simulink model "AntiBrake_model"  (R2019b)
settings: Solver=VariableStepAuto  StartTime=0.0  StopTime=20  MaxStep=0.001  RelTol=1e-3
InitFcn:
  | Cyclist_weight=85;
  | Vehicle_mass = 0.25; %Tire weight= 250g
  | gr = 9.81;
  | Wheel_Inertia = 0.0064;
  | Wheel_Radius = 0.3;
  | V=6.95; % in m/s
  | Effective_Radius_of_Disc = 0.16;
  | Coefficient_of_Brake_friction = 0.9;
  | pb=200;
  | Number_of_brake_pad = 1;
  | TB =0.01;
  | Abs=1;
libraries: simulink x1
settings Model: Creator=Avmash  LastModifiedBy=Avmash

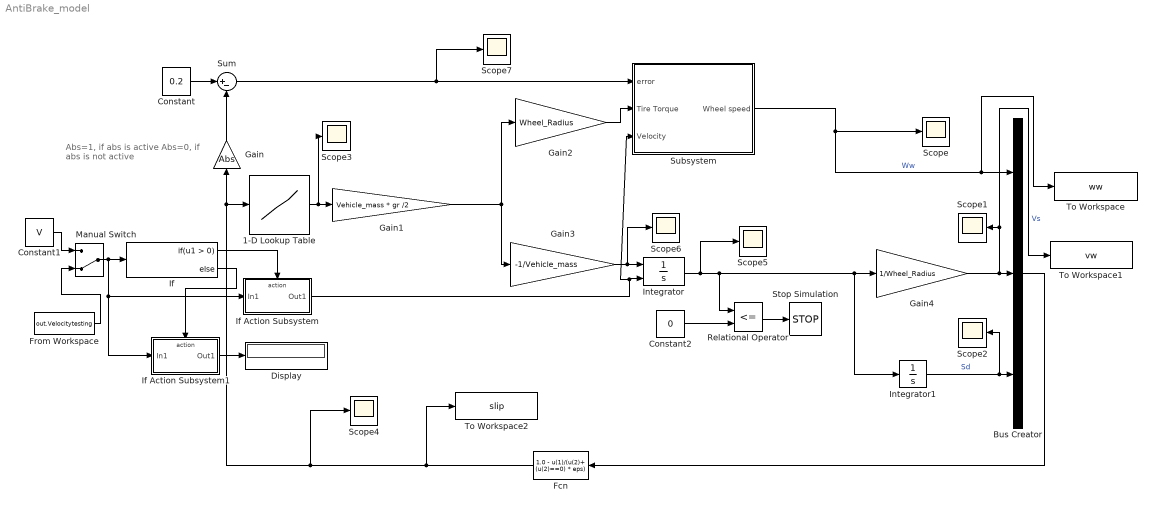
== system AntiBrake_model ==
  note: Abs=1, if abs is active
      | Abs=0, if abs is not active
  1-D Lookup Table : Lookup_n-D  NumberOfTableDimensions=1  BreakpointsForDimension1="[0\t0.0500000000000000\t0.100000000000000\t0.150000000000000\t0.200000000000000\t0.250000000000000\t0.300000000000000\t0.350000000000000\t0.400000000000000\t0.450000000000000\t0.500000000000000\t0.550000000000000\t0.600000000000000\t0.650000000000000\t0.700000000000000\t0.750000000000000\t0.800000000000000\t0.850000000000000\t0.900000000000000\t0.950000000000000\t1]"  Table="[0\t0.400000000000000\t0.800000000000000\t0.970000000000000\t1\t0.980000000000000\t0.960000000000000\t0.940000000000000\t0.920000000000000\t0.900000000000000\t0.880000000000000\t0.855000000000000\t0.830000000000000\t0.810000000000000\t0.790000000000000\t0.770000000000000\t0.750000000000000\t0.730000000000000\t0.720000000000000\t0.710000000000000\t0.700000000000000]"  InternalRulePriority=Speed  RndMeth=Simplest  InputSameDT=on
  Bus Creator : BusCreator  Inputs=3
  Constant : Constant  Value=0.2
  Constant1 : Constant  Value=V
  Constant2 : Constant  Value=0
  Display : Display
  Fcn : Fcn  Expr=1.0 - u(1)/(u(2)+ (u(2)==0) * eps)
  From Workspace : FromWorkspace  VariableName=out.Velocitytesting  SampleTime=0
  Gain : Gain  Gain=Abs
  Gain1 : Gain  Gain=Vehicle_mass * gr /2
  Gain2 : Gain  Gain=Wheel_Radius
  Gain3 : Gain  Gain=-1/Vehicle_mass
  Gain4 : Gain  Gain=1/Wheel_Radius
  If : If
  If Action Subsystem : Subsystem  TreatAsAtomicUnit=on
  If Action Subsystem1 : Subsystem  TreatAsAtomicUnit=on
  Integrator : Integrator  InitialConditionSource=external  InitialCondition=V  LimitOutput=on  UpperSaturationLimit=1000  LowerSaturationLimit=0
  Integrator1 : Integrator
  Manual Switch : ManualSwitch  CurrentSetting=0
  Relational Operator : RelationalOperator  Operator=<=  OutDataTypeStr=boolean  RndMeth=Simplest
  Scope{,1..7} (8 alike) : Scope
  Stop Simulation : Stop
  Subsystem : Subsystem
  Sum : Sum  Inputs=|+-
  To Workspace : ToWorkspace  VariableName=ww  SaveFormat=Timeseries  SampleTime=-1
  To Workspace1 : ToWorkspace  VariableName=vw  SaveFormat=Timeseries  SampleTime=-1
  To Workspace2 : ToWorkspace  VariableName=slip  SaveFormat=Timeseries  SampleTime=-1
  wires:
  1-D Lookup Table/1 -> Scope3/1, Gain1/1
  Constant/1 -> Sum/1
  Sum/1 -> Scope7/1, Subsystem/1("error ")
  Gain/1 -> Sum/2
  Fcn/1 -> To Workspace2/1, Scope4/1, 1-D Lookup Table/1, Gain/1
  Gain1/1 -> Gain3/1, Gain2/1
  Gain2/1 -> Subsystem/2(Tire Torque)
  Gain3/1 -> Scope6/1, Integrator/1
  Subsystem/1("Wheel speed ") -> Scope/1, To Workspace/1, Bus Creator/1  "Ww"
  Integrator/1 -> Scope5/1, Relational Operator/1, Integrator1/1, Gain4/1
  Integrator1/1 -> Scope2/1, Bus Creator/3  "Sd"
  Gain4/1 -> To Workspace1/1, Scope1/1, Bus Creator/2  "Vs"
  Bus Creator/1 -> Fcn/1
  Relational Operator/1 -> Stop Simulation/1
  Constant2/1 -> Relational Operator/2
  Constant1/1 -> Manual Switch/1
  If Action Subsystem/1(Out1) -> Subsystem/3(Velocity), Integrator/2
  If/1 -> If Action Subsystem/Action
  If/2 -> If Action Subsystem1/Action
  If Action Subsystem1/1(Out1) -> Display/1
  From Workspace/1 -> Manual Switch/2
  Manual Switch/1 -> If Action Subsystem/1(In1), If Action Subsystem1/1(In1), If/1

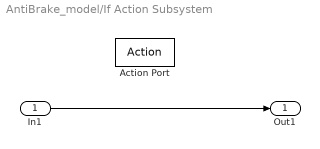
== system AntiBrake_model/If Action Subsystem ==
  In1 : Inport
  Action Port : ActionPort  ActionPortLabel=if(u1 > 0)
  Out1 : Outport
  wires:
  In1/1 -> Out1/1

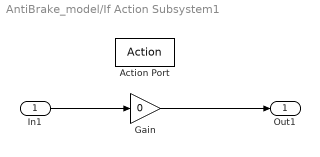
== system AntiBrake_model/If Action Subsystem1 ==
  In1 : Inport
  Action Port : ActionPort  ActionPortLabel=else
  Gain : Gain  Gain=0
  Out1 : Outport
  wires:
  In1/1 -> Gain/1
  Gain/1 -> Out1/1

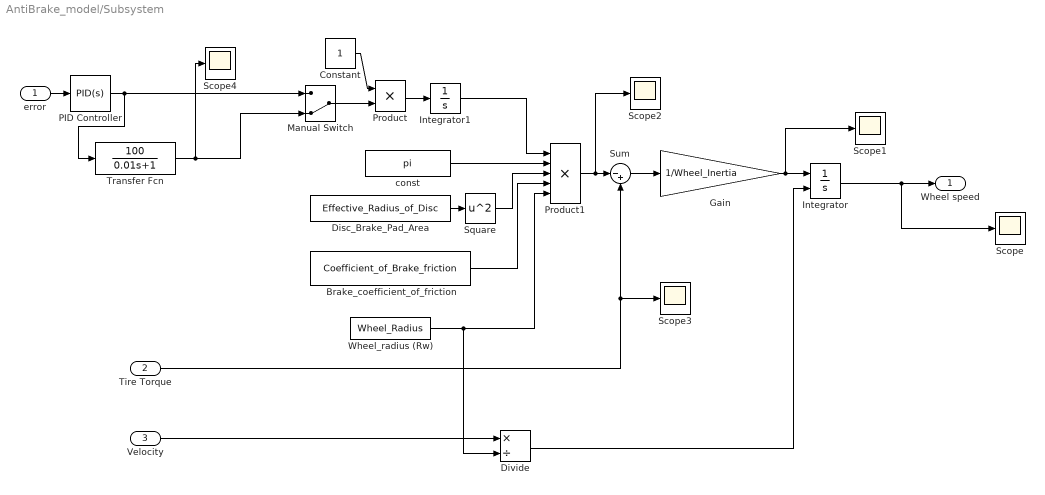
== system AntiBrake_model/Subsystem ==
  "error " : Inport
  Tire Torque : Inport  Port=2
  Velocity : Inport  Port=3
  Brake_coefficient_of_friction : Constant  Value=Coefficient_of_Brake_friction
  Constant : Constant
  Disc_Brake_Pad_Area : Constant  Value=Effective_Radius_of_Disc
  Divide : Product  Inputs=*/
  Gain : Gain  Gain=1/Wheel_Inertia
  Integrator : Integrator  InitialConditionSource=external  InitialCondition=V/Wheel_Radius  LimitOutput=on  UpperSaturationLimit=1000  LowerSaturationLimit=0
  Integrator1 : Integrator  LimitOutput=on  UpperSaturationLimit=pb
  Manual Switch : ManualSwitch  CurrentSetting=0
  PID Controller : simulink/Continuous/PID Controller  Controller=PID  Form=Parallel  TimeDomain=Continuous-time  SampleTime=-1  IntegratorMethod=Forward Euler  FilterMethod=Forward Euler  ControllerParametersSource=internal  P=22  I=4  D=0.4  UseFilter=on  N=100  TunerSelectOption=Transfer Function Based (PID Tuner App)  InitialConditionSource=internal  InitialConditionForIntegrator=0  InitialConditionForFilter=0  DifferentiatorICPrevScaledInput=0  ExternalReset=none  TrackingMode=off  Kt=1  LimitOutput=off  UpperSaturationLimit=inf  LowerSaturationLimit=-inf  LinearizeAsGain=on  AntiWindupMode=none  Kb=1  POutMin=[]  POutMax=[]  IOutMin=[]  IOutMax=[]  DOutMin=[]  DOutMax=[]  NOutMin=[]  NOutMax=[]  SumOutMin=[]  SumOutMax=[]  SaturationOutMin=[]  SaturationOutMax=[]  PParamMin=[]  PParamMax=[]  IParamMin=[]  IParamMax=[]  DParamMin=[]  DParamMax=[]  NParamMin=[]  NParamMax=[]  KbParamMin=[]  KbParamMax=[]  KtParamMin=[]  KtParamMax=[]  KbOutMin=[]  KbOutMax=[]  KtOutMin=[]  KtOutMax=[]  IntegratorOutMin=[]  IntegratorOutMax=[]  FilterOutMin=[]  FilterOutMax=[]  SumI1OutMin=[]  SumI1OutMax=[]  SumI2OutMin=[]  SumI2OutMax=[]  SumI3OutMin=[]  SumI3OutMax=[]  SumI4OutMin=[]  SumI4OutMax=[]  SumDOutMin=[]  SumDOutMax=[]  DifferentiatorOutMin=[]  DifferentiatorOutMax=[]  FilterDiffOutCoefMin=[]  FilterDiffOutCoefMax=[]  ReciprocalOutMin=[]  ReciprocalOutMax=[]  SumDenOutMin=[]  SumDenOutMax=[]  SumNumOutMin=[]  SumNumOutMax=[]  DivideOutMin=[]  DivideOutMax=[]  IntegratorContinuousStateAttributes=''  IntegratorStateMustResolveToSignalObject=off  IntegratorRTWStateStorageClass=Auto  FilterContinuousStateAttributes=''  FilterStateMustResolveToSignalObject=off  FilterRTWStateStorageClass=Auto  ParallelPVariant=InternalParameters  IdealPVariant=Disabled  IVariant=InternalParameters  DVariant=InternalParameters  IntegratorVariant=Continuous  SatVariant=Disabled  AWVariant=Passthrough  PCopyVariant=Disabled  TRVariant=Disabled  FdbkBlocksVariant=Forward  IdealPFdbkVariant=Disabled  SatFdbkVariant=Disabled  DerivativeFilterVariant=ContFilter  NVariant=InternalParameters  NCopyVariant=Disabled  FilterICVariant=InternalICsFilter  IntegratorICVariant=InternalICs  ExternalResetVariant=Disabled  TRSumVariant=Passthrough  SumFdbkVariant=Disabled  SumVariant=Sum_PID
  Product : Product
  Product1 : Product  Inputs=5
  Scope{,1..4} (5 alike) : Scope
  Square : Math  Operator=square  SaturateOnIntegerOverflow=on
  Sum : Sum  Inputs=|-+
  Transfer Fcn : TransferFcn  Numerator=[100]  Denominator=[0.01 1]
  "Wheel_radius (Rw) " : Constant  Value=Wheel_Radius
  "const " : Constant  Value=pi
  "Wheel speed " : Outport
  wires:
  "error "/1 -> PID Controller/1
  Constant/1 -> Product/1
  "const "/1 -> Product1/2
  Disc_Brake_Pad_Area/1 -> Square/1
  Square/1 -> Product1/3
  Brake_coefficient_of_friction/1 -> Product1/4
  Product1/1 -> Scope2/1, Sum/1
  Tire Torque/1 -> Scope3/1, Sum/2
  Sum/1 -> Gain/1
  Gain/1 -> Scope1/1, Integrator/1
  Manual Switch/1 -> Product/2
  PID Controller/1 -> Transfer Fcn/1, Manual Switch/1
  Product/1 -> Integrator1/1
  Integrator1/1 -> Product1/1
  Velocity/1 -> Divide/1
  Divide/1 -> Integrator/2
  "Wheel_radius (Rw) "/1 -> Divide/2, Product1/5
  Integrator/1 -> "Wheel speed "/1, Scope/1
  Transfer Fcn/1 -> Scope4/1, Manual Switch/2
